simulink model "emulacion_planta_"  (R2017b)
settings: Solver=VariableStepAuto  StartTime=0.0  StopTime=inf  FixedStep=Ts  RelTol=1e-3
undefined symbols (not defined in the file): Ts
libraries: instrumentlib x2
settings Model: Creator=Acer  LastModifiedBy=Acer
settings DataIOCC: ReturnWorkspaceOutputs=on
settings SFSimCC: SimUseLocalCustomCode=on
settings RTWCC: RTWUseLocalCustomCode=on

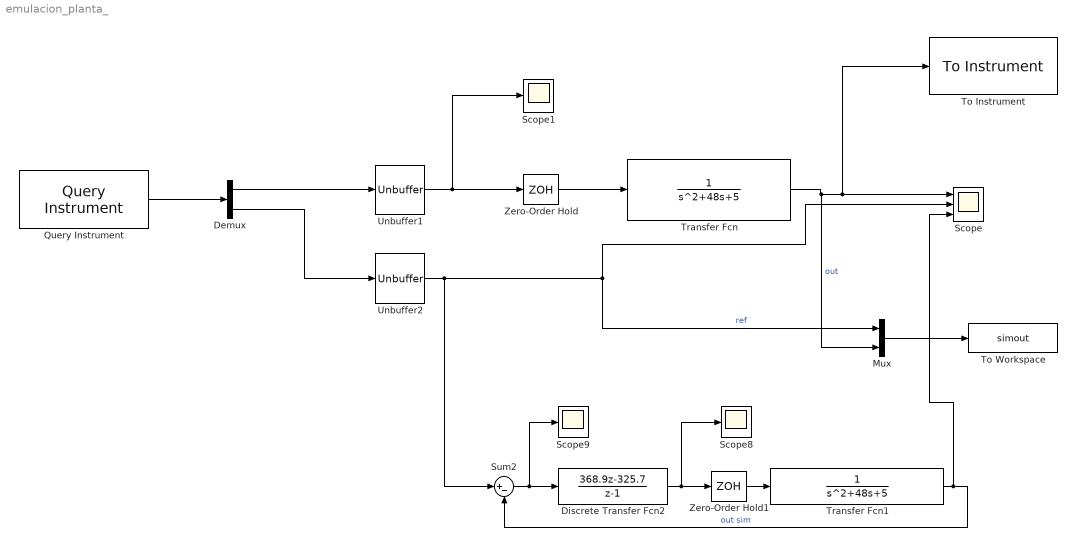
== system emulacion_planta_ ==
  Demux : Demux  Outputs=2
  Discrete Transfer Fcn2 : DiscreteTransferFcn  Numerator=[368.9 -325.7]  Denominator=[1 -1]  SampleTime=Ts
  Mux : Mux  Inputs=2
  Query Instrument : instrumentlib/Query Instrument  sampleTime=Ts  isWorkspaceObject=off  timeout=10  inputBufferSize=512  protocol=Serial  serialPort=COM3  baudRate=115200  gpibVendor=Keysight Technologies  boardIndex=0  primaryAddress=1  secondaryAddress=0  visaVendor=Keysight  visaSerialPort=0  chassisIndex=0  logicalAddress=0  tcpRemoteHost='127.0.0.1'  tcpRemotePort=4500  udpRemoteHost='127.0.0.1'  udpRemotePort=9090  visaTCPBoardIndex=0  visaTCPRemoteHost='127.0.0.1'  usbBoardIndex=0  usbManufID=0  usbModelCode=0  usbSerialNumber=0  initAction=None  initCommand='DATA:SOURCE CH1'  initFunction=get  queryCommand=''  responseFormat=ASCII  asciiFormatting='%f,%f\n'  precision=8-bit integer  byteOrder=Little endian  valuesToRead=1  removeBytes=on  afterOutputAction=Repeat query for new data  enableFrames=on  frameSize=2
      settings: SourceProductBaseCode=IC
  Scope : Scope  NumInputPorts=3
  Scope1 : Scope
  Scope8 : Scope
  Scope9 : Scope
  Sum2 : Sum  Inputs=|+-
  To Instrument : instrumentlib/To Instrument  sampleTime=-1  isWorkspaceObject=off  timeout=10  inputBufferSize=8192  protocol=Serial  serialPort=COM3  baudRate=115200  gpibVendor=ICS Electronics  boardIndex=0  primaryAddress=1  secondaryAddress=0  visaVendor=Keysight  visaSerialPort=0  chassisIndex=0  logicalAddress=0  tcpRemoteHost='127.0.0.1'  tcpRemotePort=4500  udpRemoteHost='127.0.0.1'  udpRemotePort=9090  visaTCPBoardIndex=0  visaTCPRemoteHost='127.0.0.1'  usbBoardIndex=0  usbManufID=0  usbModelCode=0  usbSerialNumber=0  initAction=None  initCommand='DATA:SOURCE CH1'  initFunction=get  command=''  sendFormat=ASCII  asciiFormatting='%5.2f\n'  precision=8-bit integer  byteOrder=Little endian
      settings: SourceProductBaseCode=IC
  To Workspace : ToWorkspace  VariableName=simout  SaveFormat=Structure With Time  SampleTime=Ts
  Transfer Fcn : TransferFcn  Denominator=[1 48 5]
  Transfer Fcn1 : TransferFcn  Denominator=[1 48 5]
  Unbuffer1 : Unbuffer
  Unbuffer2 : Unbuffer
  Zero-Order Hold : ZeroOrderHold  SampleTime=Ts
  Zero-Order Hold1 : ZeroOrderHold  SampleTime=Ts
  wires:
  Transfer Fcn/1 -> Mux/2, To Instrument/1, Scope/1  "out"
  Query Instrument/1 -> Demux/1
  Demux/1 -> Unbuffer1/1
  Demux/2 -> Unbuffer2/1
  Unbuffer2/1 -> Sum2/1, Mux/1, Scope/2  "ref"
  Unbuffer1/1 -> Zero-Order Hold/1, Scope1/1
  Mux/1 -> To Workspace/1
  Zero-Order Hold/1 -> Transfer Fcn/1
  Zero-Order Hold1/1 -> Transfer Fcn1/1
  Sum2/1 -> Discrete Transfer Fcn2/1, Scope9/1
  Transfer Fcn1/1 -> Scope/3, Sum2/2  "out sim"
  Discrete Transfer Fcn2/1 -> Zero-Order Hold1/1, Scope8/1
